simulink model "Ass1_System"  (Simulink 8.2)
settings: Solver=ode45  SolverMode=SingleTasking  StartTime=0.0  StopTime=T  RelTol=1e-3  AbsTol=1e-6
values from neighbouring files (symbols this model uses):
  dt = 1/fs    (= 0.01)    [Ass1.m]    (also in ass1_oct.m)
settings Model: Creator=schuurmans  LastModifiedBy=teodorosolises
settings DataIOCC: LimitDataPoints=off  SaveTime=off
settings OptimizationCC: BlockReduction=off  BooleanDataType=off  InitFltsAndDblsToZero=on
settings DebuggingCC: SaveWithParameterizedLinksMsg=none  SignalResolutionControl=TryResolveAllWithWarning  SolverPrmCheckMsg=none  MultiTaskDSMMsg=warning  MultiTaskCondExecSysMsg=none
settings HardwareCC: TargetUnknown=on
settings RTWCC: IncludeERTFirstTime=on
settings GRTTargetCC: TargetFcnLib=ansi_tfl_tmw.mat  ModelReferenceCompliant=off  CompOptLevelCompliant=off  MatFileLogging=off

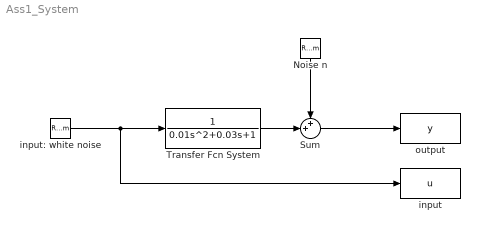
== system Ass1_System ==
  Noise n : RandomNumber  Variance=0  Seed=220  SampleTime=dt
  Sum : Sum  Inputs=++|  SaturateOnIntegerOverflow=on  InputSameDT=on  OutDataTypeStr=Inherit: Same as first input
  Transfer Fcn System : TransferFcn  Denominator=[0.01 0.03 1]
  input : ToWorkspace  VariableName=u  SampleTime=dt
      settings: Description=output
  input: white noise : RandomNumber  Seed=300  SampleTime=dt
  output : ToWorkspace  VariableName=y  SampleTime=dt
      settings: Description=output
  wires:
  Transfer Fcn System/1 -> Sum/2
  Sum/1 -> output/1
  input: white noise/1 -> Transfer Fcn System/1, input/1
  Noise n/1 -> Sum/1
